simulink model "sim_dist"  (R2016b)
settings: Solver=VariableStepAuto  StartTime=0.0  StopTime=trun  RelTol=1e-3
undefined symbols (not defined in the file): ref
libraries: cstblocks x2
settings Model: Creator=arnold  LastModifiedBy=arnold

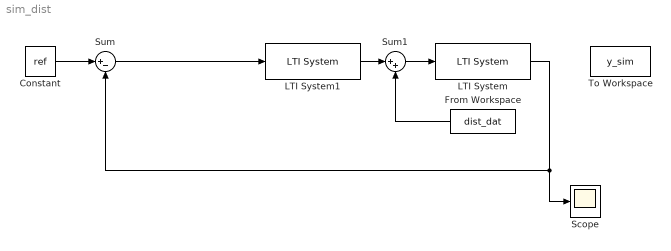
== system sim_dist ==
  Constant : Constant  Value=ref
  From Workspace : FromWorkspace  VariableName=dist_dat  SampleTime=0
  LTI System : cstblocks/LTI System  sys=G  IC=[]
  LTI System1 : cstblocks/LTI System  sys=Di  IC=[]
  Scope : Scope
  Sum : Sum  Inputs=|+-
  Sum1 : Sum  Inputs=|++
  To Workspace : ToWorkspace  VariableName=y_sim  SaveFormat=Timeseries  SampleTime=-1
  wires:
  Sum/1 -> LTI System1/1
  LTI System/1 -> Scope/1, Sum/2
  From Workspace/1 -> Sum1/2
  Constant/1 -> Sum/1
  LTI System1/1 -> Sum1/1
  Sum1/1 -> LTI System/1
